simulink model "PROBLEM_8_LIFT_MODEL"  (R2020b)
settings: Solver=VariableStepAuto  StartTime=0.0  StopTime=10.0  RelTol=1e-3
settings Model: Creator=intel  LastModifiedBy=intel

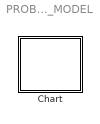
== system PROBLEM_8_LIFT_MODEL ==
  Chart : Stateflow chart  TreatAsAtomicUnit=on

== stateflow chart PROBLEM_8_LIFT_MODEL/Chart ==
  state Preparing1 to Move Down
    state Door Closing to Move Down
    state Elevator1
      Starting Down
  state Preparing to Moving Up
    state Door Closing to Move Upe
    state Elevator1
      Starting Up
  state Elevator Idle
  state Elevator1 Moving
  (default) -> Elevator Idle
